simulink model "GFM_MMC"  (R2021a)
settings: Solver=ode23tb  StartTime=0.0  StopTime=3  MaxStep=1e-4  RelTol=1e-3
libraries: GFM_Lib x1, Source_Lib x1, spspowerguiLib x1
settings Model: Creator=Frederic_Colas  LastModifiedBy=Frederic_Colas

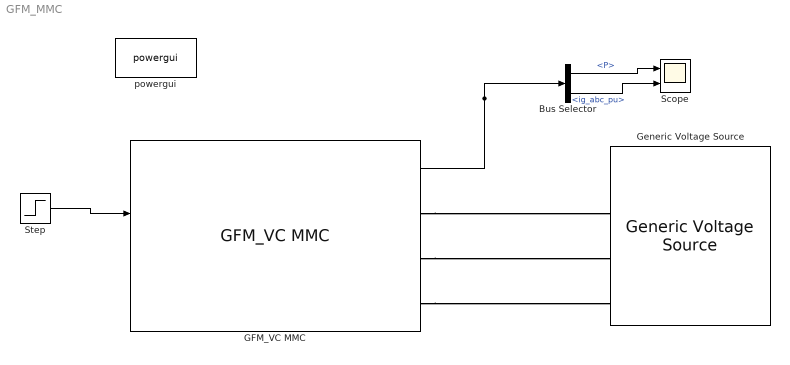
== system GFM_MMC ==
  Bus Selector : BusSelector  OutputSignals=P,I.ig_abc_pu
  GFM_VC MMC : GFM_Lib/GFM_VC MMC  fn=50  Sn=1000e6  Pn=1000e6  Udcn=640e3  Output_Delay=100e-6  Un1=320e3  Un2=400e3  Rt_pu=0.005  Lt_pu=0.15  Lm_pu=500  Rm_pu=500  Larm_pu=0.18  Rarm_pu=0.005  nSM=0  Hc=40  DC_source=on  wn_PLL=500  zeta_PLL=1  Val_Freq_Support=off  R_percent=4  Lc_eq=0.15+0.18/2  Rv=0.09  W_TVR=60  I_max_pu=1.2  Tr_I_max=10  I_Max_TVI_pu=1.2  DX_DR=5  MMC_Control_Type=Energy Based  Diff_CC_fn=200  Diff_CC_zeta=1  fn_Wtot=5  zeta_Wtot=1  fn_Wdiff=3  zeta_Wdiff=1  Advanced=on  gainpopup=With Inertia  f_Inertia_Less=5  zeta_Inertia_Less=1  Tr_Inertia_Less=100  Param_Inertia=PI  H_GFo=5  zeta_GFo=0.7  LFpopup=PQ  P0=0.2  Q0=0  V0=1  Theta0=0
      settings: SourceProductName=VSC4SPS
  Generic Voltage Source : Source_Lib/Generic Voltage Source  SourceNature_str=INFINITE  fn=50  Sn=1e9  Un=400e3  Time_Step=25e-6  LFpopup=Swing  P0=-491545376.7896  Q0=82825649.5509  V0_pu=1  U0=20000  Theta0_deg=0  H_s=5  DroopOnOff=on  R_percent=4  TN=1  TD=2
      settings: SourceProductName=VSC4SPS
  Scope : Scope  NumInputPorts=2
  Step : Step  After=0.4  SampleTime=0
  powergui : spspowerguiLib/powergui  Priority=1  SimulationMode=Discrete  SampleTime=25e-6  frequency=60  Iterations=50  frequencyindice=50  Pbase=100e6  ErrMax=1e-4  UnitsV=kV  UnitsW=MW  buscounter=0  FunctionMessages=off  echomessages=off  EnableUseOfTLC=off  CurrentSourceSwitches=off  DisableSnubberDevices=off  DisableRonSwitches=off  DisableVfSwitches=off  DisplayEquations=off  AutomaticDiscreteSolvers=off  SolverType=Tustin/Backward Euler (TBE)  Interpol=off  ExternalGateDelay=off  methode=off  Ts=100  x0status=blocks  SPID=on  SwTol=0  HookPort=off  NonlinearTolerance=1e-4  nMaxIteration=100  ContinueOnMaxIteration=off  RestoreLinks=warning  ResistiveCurrentMeasurement=off  Frange=[0:2:500]  Ylog=off  Xlog=on  ShowGrid=off  save=off  variable=ZData  structure=0  ZoomFFT=off  StartTime=0.0  cycles=1  DisplayStyle=1  fundamental=60  FreqAxis=off  MaxFrequency=1000  frequencyindicesteady=1  RmsSteady=1  display=off
  wires:
  Step/1 -> GFM_VC MMC/2
  GFM_VC MMC/1 -> Bus Selector/1
  Bus Selector/1 -> Scope/1  "<P>"
  Bus Selector/2 -> Scope/2  "<ig_abc_pu>"
  connections:
  GFM_VC MMC/RConn1 -- Generic Voltage Source/RConn1
  GFM_VC MMC/RConn2 -- Generic Voltage Source/RConn2
  GFM_VC MMC/RConn3 -- Generic Voltage Source/RConn3
